simulink model "BBBCSystem"  (R2023b)
settings: Solver=ode3  StartTime=0.0  StopTime=25  FixedStep=0.01  RelTol=1e-3  EnableMultiTasking=on
values from neighbouring files (symbols this model uses):
  Kc = 0.02    [dataset.mat]    (also in initiateVars.m; system_workspace.mat; system_workspace_ayk.mat)
  Kd = x(i,2)    [BCostPD.m]    (also in dataset.mat = 2; initiateVars.m = 2; system_workspace.mat = 2; system_workspace_ayk.mat = 2)
undefined symbols (not defined in the file or in its folder): Ki, magnitude
libraries: simulink x1
settings Model: Creator=fd  LastModifiedBy=fethi
settings SolverCC: AlgebraicLoopSolver=TrustRegion
settings DataIOCC: LimitDataPoints=on  SaveFormat=Array  SignalLoggingSaveFormat=ModelDataLogs  ReturnWorkspaceOutputs=off
settings OptimizationCC: ExpressionDepthLimit=2147483647  LifeSpan=inf
settings DebuggingCC: UnderspecifiedInitializationDetection=Classic  MergeDetectMultiDrivingBlocksExec=none  SolverPrmCheckMsg=warning  MultiTaskDSMMsg=warning  MultiTaskCondExecSysMsg=none  FcnCallInpInsideContextMsg=warning  UnconnectedInputMsg=warning  UnconnectedOutputMsg=warning  UnconnectedLineMsg=warning  StateNameClashWarn=warning  SFUnexpectedBacktrackingDiag=warning  SFNoUnconditionalDefaultTransitionDiag=warning  SFExecutionAtInitializationDiag=none  ArithmeticOperatorsInVariantConditions=warning
settings HardwareCC: ProdBitPerPointer=32  ProdBitPerSizeT=32  ProdBitPerPtrDiffT=32  ProdLargestAtomicFloat=None  ProdIntDivRoundTo=Undefined  ProdEndianess=Unspecified  ProdWordSize=32  ProdHWDeviceType=32-bit Generic
settings ModelReferenceCC: PropagateSignalLabelsOutOfModel=off
settings SFSimCC: SimUseLocalCustomCode=off  CustomCodeUndefinedFunction=UseInterfaceOnly
settings RTWCC: RTWUseLocalCustomCode=off
settings CodeAppCC: StateflowObjectComments=on
settings GRTTargetCC: TargetLangStandard=C89/C90 (ANSI)  CombineOutputUpdateFcns=off  GRTInterface=on
settings ConfigComp: CovMetricSettings=dw  CovSaveCumulativeToWorkspaceVar=on  CovSaveSingleToWorkspaceVar=on  CovExternalEMLEnable=off

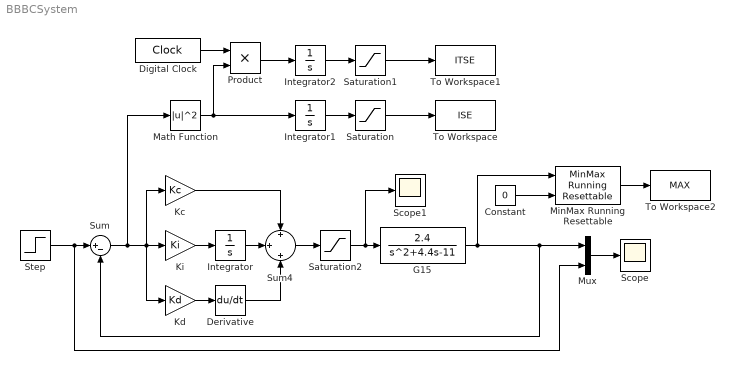
== system BBBCSystem ==
  Constant : Constant  Value=0
  Derivative : Derivative
  Digital Clock : DigitalClock  SampleTime=0.01
  "G15 " : TransferFcn  Numerator=[2.4]  Denominator=[1 4.4 -11]
  Integrator : Integrator
  Integrator1 : Integrator
  Integrator2 : Integrator
  Kc : Gain  Gain=Kc
  Kd : Gain  Gain=Kd
  Ki : Gain  Gain=Ki
  Math Function : Math  Operator=magnitude^2  SignedPower=on
  MinMax Running Resettable : simulink/Math Operations/MinMax Running Resettable  Function=max  vinit=0
  Mux : Mux  Inputs=2
  Product : Product  RndMeth=Zero
  Saturation : Saturate  UpperLimit=800
  Saturation1 : Saturate  UpperLimit=800
  Saturation2 : Saturate  UpperLimit=100  LowerLimit=-100
  Scope : Scope
  Scope1 : Scope
  Step : Step  Time=0  SampleTime=0.01
  Sum : Sum  Inputs=|+-
  Sum4 : Sum  Inputs=+|+|+
  To Workspace : ToWorkspace  VariableName=ISE  SampleTime=-1
  To Workspace1 : ToWorkspace  VariableName=ITSE  SampleTime=-1
  To Workspace2 : ToWorkspace  VariableName=MAX  SampleTime=-1
  wires:
  Step/1 -> Mux/2, Sum/1
  Integrator1/1 -> Saturation/1
  Math Function/1 -> Product/2, Integrator1/1
  Saturation/1 -> To Workspace/1
  Kc/1 -> Sum4/1
  Integrator/1 -> Sum4/2
  Ki/1 -> Integrator/1
  Mux/1 -> Scope/1
  Digital Clock/1 -> Product/1
  Product/1 -> Integrator2/1
  Integrator2/1 -> Saturation1/1
  Saturation1/1 -> To Workspace1/1
  "G15 "/1 -> Sum/2, Mux/1, MinMax Running Resettable/1
  MinMax Running Resettable/1 -> To Workspace2/1
  Constant/1 -> MinMax Running Resettable/2
  Sum/1 -> Math Function/1, Kd/1, Ki/1, Kc/1
  Kd/1 -> Derivative/1
  Derivative/1 -> Sum4/3
  Saturation2/1 -> Scope1/1, "G15 "/1
  Sum4/1 -> Saturation2/1
